simulink model "simPgenH2Hinf"  (R2016a)
settings: Solver=VariableStepAuto  StartTime=0.0  StopTime=40  RelTol=1e-3
values from neighbouring files (symbols this model uses):
  Ksinf = minreal(ss(Ainf,Zinf*Linf,-Finf,0))    [exercise_class18.m]
  nd = nx    [exercise_class18.m]
  nn = ny    [exercise_class18.m]
  nu = size(BG,2)    [exercise_class18.m]
  nw = nd+nn    [exercise_class18.m]
  ny = size(CG,1)    [exercise_class18.m]
  nz = nz1+nz2    [exercise_class18.m]
  nz1 = nx    [exercise_class18.m]
  nz2 = nu    [exercise_class18.m]
  Ps = ss(AP,BP,CP,DP)    [exercise_class18.m]
  sqrtQ = chol(Q)    [exercise_class18.m]
  sqrtR = chol(R)    [exercise_class18.m]
  sqrtRd = chol(Rd)    [exercise_class18.m]
  sqrtRn = chol(Rn)    [exercise_class18.m]
  x0 = [1 3 7 -1 0 1]'    [exercise_class18.m]
undefined symbols (not defined in the file or in its folder): Ks
libraries: simulink x2
settings Model: Creator=rafae  LastModifiedBy=rafae

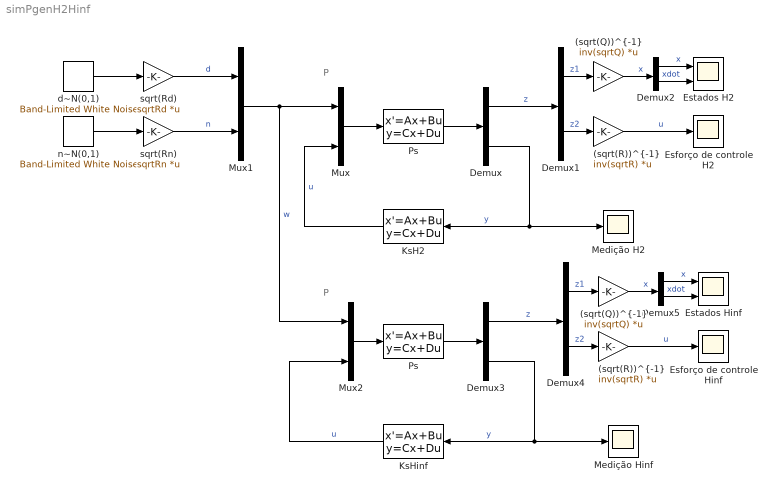
== system simPgenH2Hinf ==
  note: P
  note: P
  "(sqrt(Q))^{-1}" : Gain  Gain=inv(sqrtQ)  Multiplication=Matrix(K*u)
  "(sqrt(Q))^{-1} " : Gain  Gain=inv(sqrtQ)  Multiplication=Matrix(K*u)
  "(sqrt(R))^{-1} " : Gain  Gain=inv(sqrtR)  Multiplication=Matrix(K*u)
  "(sqrt(R))^{-1} " : Gain  Gain=inv(sqrtR)  Multiplication=Matrix(K*u)
  Demux : Demux  Outputs=[nz ny]
  Demux1 : Demux  Outputs=[nz1 nz2]
  Demux2 : Demux  Outputs=[3 3]
  Demux3 : Demux  Outputs=[nz ny]
  Demux4 : Demux  Outputs=[nz1 nz2]
  Demux5 : Demux  Outputs=[3 3]
  Esforço de controle H2 : Scope
  Esforço de controle Hinf : Scope
  Estados H2 : Scope  NumInputPorts=2
  Estados Hinf : Scope  NumInputPorts=2
  KsH2 : StateSpace  A=Ks.A  B=Ks.B  C=Ks.C  D=Ks.D  X0=0
  KsHinf : StateSpace  A=Ksinf.A  B=Ksinf.B  C=Ksinf.C  D=Ksinf.D  X0=0
  Medição H2 : Scope
  Medição Hinf : Scope
  Mux : Mux  Inputs=[nw nu]
  Mux1 : Mux  Inputs=[nd nn]
  Mux2 : Mux  Inputs=[nw nu]
  Ps : StateSpace  A=Ps.A  B=Ps.B  C=Ps.C  D=Ps.D  X0=x0
  "Ps " : StateSpace  A=Ps.A  B=Ps.B  C=Ps.C  D=Ps.D  X0=x0
  d~N(0,1) : simulink/Sources/Band-Limited White Noise  Cov=[0.001 0.001 0.001 0.001 0.001 0.001]  Ts=0.001  seed=[23341]
  n~N(0,1) : simulink/Sources/Band-Limited White Noise  Cov=[0.001 0.001 0.001]  Ts=0.001  seed=[23341]
  sqrt(Rd) : Gain  Gain=sqrtRd  Multiplication=Matrix(K*u)
  sqrt(Rn) : Gain  Gain=sqrtRn  Multiplication=Matrix(K*u)
  wires:
  Mux/1 -> Ps/1
  Ps/1 -> Demux/1
  Demux/2 -> KsH2/1, Medição H2/1  "y"
  KsH2/1 -> Mux/2  "u"
  d~N(0,1)/1 -> sqrt(Rd)/1
  n~N(0,1)/1 -> sqrt(Rn)/1
  sqrt(Rn)/1 -> Mux1/2  "n"
  Demux/1 -> Demux1/1  "z"
  Demux1/1 -> "(sqrt(Q))^{-1}"/1  "z1"
  Demux1/2 -> "(sqrt(R))^{-1} "/1  "z2"
  "(sqrt(R))^{-1} "/1 -> Esforço de controle H2/1  "u"
  "(sqrt(Q))^{-1}"/1 -> Demux2/1  "x"
  Demux2/1 -> Estados H2/1  "x"
  Demux2/2 -> Estados H2/2  "xdot"
  Mux2/1 -> "Ps "/1
  "Ps "/1 -> Demux3/1
  Demux3/2 -> KsHinf/1, Medição Hinf/1  "y"
  sqrt(Rd)/1 -> Mux1/1  "d"
  Demux3/1 -> Demux4/1  "z"
  Demux4/1 -> "(sqrt(Q))^{-1} "/1  "z1"
  Demux4/2 -> "(sqrt(R))^{-1} "/1  "z2"
  "(sqrt(R))^{-1} "/1 -> Esforço de controle Hinf/1  "u"
  "(sqrt(Q))^{-1} "/1 -> Demux5/1  "x"
  Demux5/1 -> Estados Hinf/1  "x"
  Demux5/2 -> Estados Hinf/2  "xdot"
  KsHinf/1 -> Mux2/2  "u"
  Mux1/1 -> Mux2/1, Mux/1  "w"
